simulink model "Subsystem"  (R2020a)
settings: Solver=FixedStepAuto  StartTime=0.0  StopTime=10.0  FixedStep=0.2  RelTol=1e-3
settings Model: Creator=anjal  LastModifiedBy=anjal
settings DataIOCC: SaveOutput=off  SaveTime=off

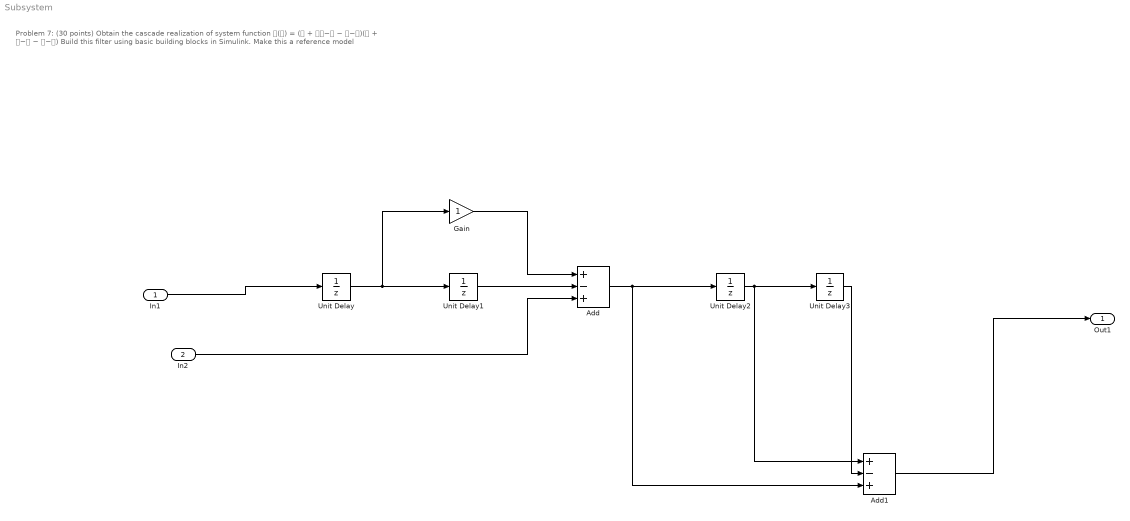
== system Subsystem ==
  note: Problem 7: (30 points) Obtain the cascade realization of system function
      | 𝐇(𝐳) = (𝟏 + 𝟐𝐳−𝟏 − 𝐳−𝟐)(𝟏 + 𝐳−𝟏 − 𝐳−𝟐)
      | Build this filter using basic building blocks in Simulink. Make this a reference model
  In1 : Inport  OutDataTypeStr=double  PortDimensions=1  SampleTime=[0.20000000000000001,0]
  In2 : Inport  Port=2  OutDataTypeStr=double  PortDimensions=1  SampleTime=[0.20000000000000001,0]
  Add : Sum  Inputs=+-+
  Add1 : Sum  Inputs=+-+
  Gain : Gain
  Unit Delay{,1..3} (4 alike) : UnitDelay  SampleTime=-1  HasFrameUpgradeWarning=on
  Out1 : Outport  OutDataTypeStr=double  PortDimensions=1  SampleTime=[0.20000000000000001,0]
  wires:
  Unit Delay/1 -> Unit Delay1/1, Gain/1
  Unit Delay1/1 -> Add/2
  Unit Delay2/1 -> Add1/1, Unit Delay3/1
  In1/1 -> Unit Delay/1
  Gain/1 -> Add/1
  In2/1 -> Add/3
  Unit Delay3/1 -> Add1/2
  Add1/1 -> Out1/1
  Add/1 -> Add1/3, Unit Delay2/1
